simulink model "Pendulum_Oscillator"  (R2024a)
settings: Solver=VariableStepAuto  StartTime=0.0  StopTime=10  MaxStep=0.01  RelTol=1e-3
model workspace (MAT data in the model file):
  I0 = 0.088
  L = 0.43
  g = 9.81
  m = 1
settings Model: Creator=91839
settings SolverCC: AlgebraicLoopSolver=TrustRegion
settings DataIOCC: ExternalInput=data  LoadExternalInput=on  SaveFormat=Array  DSMLogging=off  ReturnWorkspaceOutputs=off
settings DebuggingCC: UnconnectedInputMsg=warning  UnconnectedOutputMsg=warning  UnconnectedLineMsg=warning
settings ModelReferenceCC: EnableRefExpFcnMdlSchedulingChecks=on
settings SFSimCC: CustomCodeUndefinedFunction=UseInterfaceOnly
settings RTWCC: GPUComputeCapability=3.5

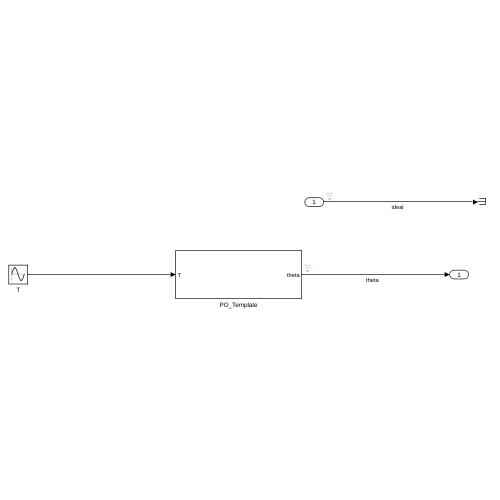
[thumbnail: Simulink's stored preview of the top-level diagram]
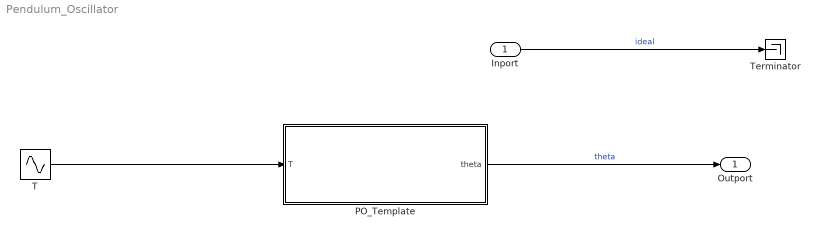
== system Pendulum_Oscillator ==
  Inport : Inport
  PO_Template : Subsystem
  T : Sin  SampleTime=0
  Terminator : Terminator
  Outport : Outport
  wires:
  Inport/1 -> Terminator/1  "ideal"
  T/1 -> PO_Template/1(T)
  PO_Template/1(theta) -> Outport/1  "theta"

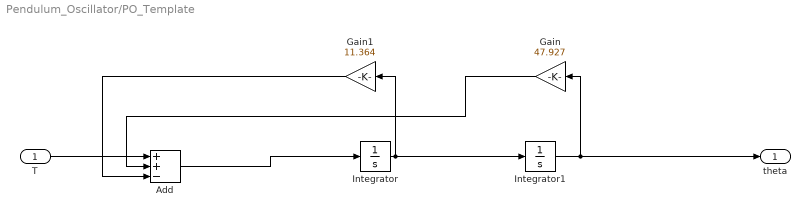
== system Pendulum_Oscillator/PO_Template ==
  T : Inport
  Add : Sum  Inputs=++-
  Gain : Gain  Gain=47.927
  Gain1 : Gain  Gain=11.364
  Integrator : Integrator
  Integrator1 : Integrator
  theta : Outport
  wires:
  Integrator/1 -> Gain1/1, Integrator1/1
  T/1 -> Add/1
  Integrator1/1 -> Gain/1, theta/1
  Add/1 -> Integrator/1
  Gain/1 -> Add/2
  Gain1/1 -> Add/3
